simulink model "verify_Ground_Storage_mdl"  (R2016b)
settings: Solver=ode113  StartTime=0  StopTime=24*3600  MaxStep=600  RelTol=1e-3  EnableMultiTasking=on
InitFcn:
  | load('DE_TRY2010_13_averageYear')
libraries: carnot x7
settings Model: Creator=drhf  LastModifiedBy=User
settings DataIOCC: SaveFormat=Array  SignalLoggingSaveFormat=ModelDataLogs
settings OptimizationCC: ExpressionDepthLimit=2147483647  LifeSpan=inf
settings DebuggingCC: UnderspecifiedInitializationDetection=Classic  MergeDetectMultiDrivingBlocksExec=none  SolverPrmCheckMsg=warning  FcnCallInpInsideContextMsg=warning  StateNameClashWarn=warning  SFUnexpectedBacktrackingDiag=warning  SFNoUnconditionalDefaultTransitionDiag=warning  SFExecutionAtInitializationDiag=none
settings HardwareCC: ProdBitPerPointer=32  ProdBitPerSizeT=32  ProdBitPerPtrDiffT=32  ProdLargestAtomicFloat=None  ProdIntDivRoundTo=Undefined  ProdEndianess=Unspecified  ProdWordSize=32  ProdHWDeviceType=32-bit Generic
settings ModelReferenceCC: PropagateSignalLabelsOutOfModel=off
settings GRTTargetCC: TargetLangStandard=C89/C90 (ANSI)  GeneratePreprocessorConditionals=Disable all  CombineOutputUpdateFcns=off  GRTInterface=on
settings ConfigComp: CovMetricSettings=dw  CovHtmlReporting=on  CovSaveCumulativeToWorkspaceVar=on  CovSaveSingleToWorkspaceVar=on  CovExternalEMLEnable=off

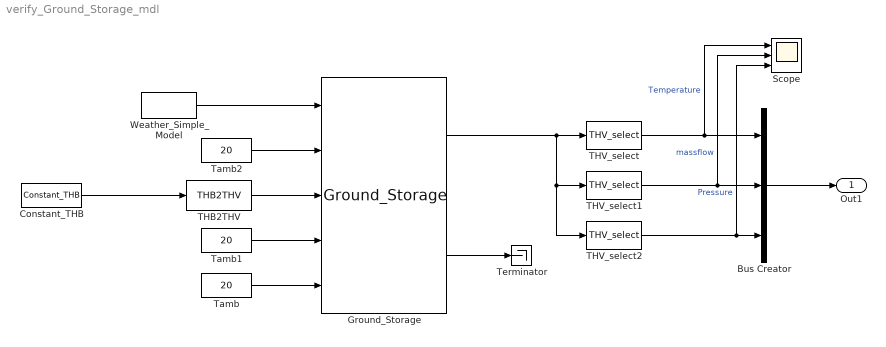
== system verify_Ground_Storage_mdl ==
  Bus Creator : BusCreator  Inputs=3
  Constant_THB : carnot/Source/Simple/Constant_THB  t=40  mdot=0.2  p=1e5  mID=No Pressure Drop  fluid=Water  mix=0  mix2=0  mix3=0  dia=0.02  hgt=0
  Ground_Storage : carnot/Storage/Thermal/Ground_Storage  xs=10  ys=10  zs=5  ground=clay (humid)  fill=clay (humid)  dp=0.1  kp=0.001  zp=1  np=20  t0=20  refine=1  mpts=5
  Scope : Scope  NumInputPorts=3
  THB2THV : carnot/Toolbox/THB2THV
  THV_select : carnot/Outputs/THV_select  f=off  t=on  m=off  p=off  id=off  mix=off  d=off  dpcon=off  dplin=off  dpqua=off
  THV_select1 : carnot/Outputs/THV_select  f=off  t=off  m=on  p=off  id=off  mix=off  d=off  dpcon=off  dplin=off  dpqua=off
  THV_select2 : carnot/Outputs/THV_select  f=off  t=off  m=off  p=on  id=off  mix=off  d=off  dpcon=off  dplin=off  dpqua=off
  Tamb : Constant  Value=20
  Tamb1 : Constant  Value=20
  Tamb2 : Constant  Value=20
  Terminator : Terminator
  Weather_Simple_Model : carnot/Weather/Weather_Simple_Model  lat=60  Ibn=900  Idg=100  tamb=5  deltaTsky=-6  rh=50  precip="10e-3/24/3600           % 10 mm in 24 h"  cloud=0.125  p=1013e2  vw=1  wdir=270
  Out1 : Outport
  wires:
  Bus Creator/1 -> Out1/1
  Tamb/1 -> Ground_Storage/5
  THB2THV/1 -> Ground_Storage/3
  Ground_Storage/1 -> THV_select2/1, THV_select1/1, THV_select/1
  Tamb1/1 -> Ground_Storage/4
  Tamb2/1 -> Ground_Storage/2
  Weather_Simple_Model/1 -> Ground_Storage/1
  Constant_THB/1 -> THB2THV/1
  Ground_Storage/2 -> Terminator/1
  THV_select/1 -> Scope/1, Bus Creator/1  "Temperature"
  THV_select1/1 -> Scope/2, Bus Creator/2  "massflow"
  THV_select2/1 -> Scope/3, Bus Creator/3  "Pressure"
